simulink model "quad_new_leg_raibert_strategy_v2"  (R2018a)
settings: Solver=ode15s  StartTime=0.0  StopTime=10.0  RelTol=1e-3
values from neighbouring files (symbols this model uses):
  X = ([-L/2, L/2, L/2, -L/2])    [draw_cube.m]
  Y = ([-W/2, -W/2, W/2, W/2])    [draw_cube.m]
undefined symbols (not defined in the file or in its folder): body, ctrl, ground, planner, Z
libraries: nesl_utility x73, sm_lib x41, simulink x29, Contact_Forces_Lib x4, Parts_Lib x4, sharedtransform x1, dspstat3 x1
(part 4 of 4)

== system quad_new_leg_raibert_strategy_v2/leg_rl/u_joint_ctrl  ==
  tgt_angle : Inport
  has_ctrl : Inport  Port=2
  PID Controller : simulink/Continuous/PID Controller  Controller=PID  TimeDomain=Continuous-time  SampleTime=-1  IntegratorMethod=Forward Euler  FilterMethod=Forward Euler  Form=Parallel  UseFilter=on  ControllerParametersSource=internal  P=ctrl.pos_kp  I=ctrl.pos_ki  D=ctrl.pos_kd  N=100  InitialConditionSource=internal  InitialConditionForIntegrator=0  InitialConditionForFilter=0  ExternalReset=none  LimitOutput=off  UpperSaturationLimit=inf  LowerSaturationLimit=-inf  LinearizeAsGain=on  AntiWindupMode=none  Kb=1  TrackingMode=off  Kt=1  PParamMin=[]  PParamMax=[]  IParamMin=[]  IParamMax=[]  DParamMin=[]  DParamMax=[]  NParamMin=[]  NParamMax=[]  KbParamMin=[]  KbParamMax=[]  KtParamMin=[]  KtParamMax=[]  POutMin=[]  POutMax=[]  IOutMin=[]  IOutMax=[]  DOutMin=[]  DOutMax=[]  NOutMin=[]  NOutMax=[]  KbOutMin=[]  KbOutMax=[]  KtOutMin=[]  KtOutMax=[]  IntegratorOutMin=[]  IntegratorOutMax=[]  FilterOutMin=[]  FilterOutMax=[]  SumOutMin=[]  SumOutMax=[]  SumI1OutMin=[]  SumI1OutMax=[]  SumI2OutMin=[]  SumI2OutMax=[]  SumI3OutMin=[]  SumI3OutMax=[]  SumDOutMin=[]  SumDOutMax=[]  SaturationOutMin=[]  SaturationOutMax=[]  IntegratorContinuousStateAttributes=''  IntegratorStateMustResolveToSignalObject=off  IntegratorRTWStateStorageClass=Auto  FilterContinuousStateAttributes=''  FilterStateMustResolveToSignalObject=off  FilterRTWStateStorageClass=Auto  DifferentiatorICPrevScaledInput=0  DifferentiatorOutMin=[]  DifferentiatorOutMax=[]  FilterDiffOutCoefMin=[]  FilterDiffOutCoefMax=[]  SumDenOutMin=[]  SumDenOutMax=[]  SumNumOutMin=[]  SumNumOutMax=[]  ReciprocalOutMin=[]  ReciprocalOutMax=[]  DivideOutMin=[]  DivideOutMax=[]  TunerSelectOption=Transfer Function Based (PID Tuner App)
  PID Controller3 : simulink/Continuous/PID Controller  Controller=PID  TimeDomain=Continuous-time  SampleTime=-1  IntegratorMethod=Forward Euler  FilterMethod=Forward Euler  Form=Parallel  UseFilter=on  ControllerParametersSource=internal  P=ctrl.vel_kp  I=ctrl.vel_ki  D=ctrl.vel_kd  N=100  InitialConditionSource=internal  InitialConditionForIntegrator=0  InitialConditionForFilter=0  ExternalReset=none  LimitOutput=off  UpperSaturationLimit=inf  LowerSaturationLimit=-inf  LinearizeAsGain=on  AntiWindupMode=none  Kb=1  TrackingMode=off  Kt=1  PParamMin=[]  PParamMax=[]  IParamMin=[]  IParamMax=[]  DParamMin=[]  DParamMax=[]  NParamMin=[]  NParamMax=[]  KbParamMin=[]  KbParamMax=[]  KtParamMin=[]  KtParamMax=[]  POutMin=[]  POutMax=[]  IOutMin=[]  IOutMax=[]  DOutMin=[]  DOutMax=[]  NOutMin=[]  NOutMax=[]  KbOutMin=[]  KbOutMax=[]  KtOutMin=[]  KtOutMax=[]  IntegratorOutMin=[]  IntegratorOutMax=[]  FilterOutMin=[]  FilterOutMax=[]  SumOutMin=[]  SumOutMax=[]  SumI1OutMin=[]  SumI1OutMax=[]  SumI2OutMin=[]  SumI2OutMax=[]  SumI3OutMin=[]  SumI3OutMax=[]  SumDOutMin=[]  SumDOutMax=[]  SaturationOutMin=[]  SaturationOutMax=[]  IntegratorContinuousStateAttributes=''  IntegratorStateMustResolveToSignalObject=off  IntegratorRTWStateStorageClass=Auto  FilterContinuousStateAttributes=''  FilterStateMustResolveToSignalObject=off  FilterRTWStateStorageClass=Auto  DifferentiatorICPrevScaledInput=0  DifferentiatorOutMin=[]  DifferentiatorOutMax=[]  FilterDiffOutCoefMin=[]  FilterDiffOutCoefMax=[]  SumDenOutMin=[]  SumDenOutMax=[]  SumNumOutMin=[]  SumNumOutMax=[]  ReciprocalOutMin=[]  ReciprocalOutMax=[]  DivideOutMin=[]  DivideOutMax=[]  TunerSelectOption=Transfer Function Based (PID Tuner App)
  PSConv3 : nesl_utility/PS-Simulink Converter  PhysicalDomain=network_engine_domain  SubClassName=ps_output  LeftPortType=input  RightPortType=output  PseudoPeriodic=off  Frequencies=[]  Unit=1  AffineConversion=off
  PSConv4 : nesl_utility/PS-Simulink Converter  PhysicalDomain=network_engine_domain  SubClassName=ps_output  LeftPortType=input  RightPortType=output  PseudoPeriodic=off  Frequencies=[]  Unit=1  AffineConversion=off
  Product : Product
  SPConv : nesl_utility/Simulink-PS Converter  PhysicalDomain=network_engine_domain  SubClassName=ps_input  LeftPortType=input  RightPortType=output  PseudoPeriodic=off  Frequencies=[]  NoiseDistribution=none  NoiseParameters=[]  Unit=1  AffineConversion=off  FilteringAndDerivatives=filter  SimscapeFilterOrder=2  InputFilterTimeConstant=0.001  UdotUserProvided=1
  Sum1 : Sum  Inputs=|+-
  Sum6 : Sum  Inputs=|+-
  curr_angle : PMIOPort  Side=Left
  curr_omega : PMIOPort  Port=2  Side=Left
  torque : PMIOPort  Port=3  Side=Right
  wires:
  tgt_angle/1 -> Sum1/1
  Sum1/1 -> PID Controller/1
  PID Controller/1 -> Sum6/1
  Sum6/1 -> PID Controller3/1
  Product/1 -> SPConv/1
  PSConv3/1 -> Sum1/2
  has_ctrl/1 -> Product/1
  PID Controller3/1 -> Product/2
  PSConv4/1 -> Sum6/2
  connections:
  PSConv3/LConn1 -- curr_angle/RConn1
  SPConv/RConn1 -- torque/RConn1
  curr_omega/RConn1 -- PSConv4/LConn1

== system quad_new_leg_raibert_strategy_v2/leg_rr/k_joint_ctrl ==
  tgt_angle : Inport
  has_ctrl : Inport  Port=2
  PID Controller : simulink/Continuous/PID Controller  Controller=PID  TimeDomain=Continuous-time  SampleTime=-1  IntegratorMethod=Forward Euler  FilterMethod=Forward Euler  Form=Parallel  UseFilter=on  ControllerParametersSource=internal  P=ctrl.pos_kp  I=ctrl.pos_ki  D=ctrl.pos_kd  N=100  InitialConditionSource=internal  InitialConditionForIntegrator=0  InitialConditionForFilter=0  ExternalReset=none  LimitOutput=off  UpperSaturationLimit=inf  LowerSaturationLimit=-inf  LinearizeAsGain=on  AntiWindupMode=none  Kb=1  TrackingMode=off  Kt=1  PParamMin=[]  PParamMax=[]  IParamMin=[]  IParamMax=[]  DParamMin=[]  DParamMax=[]  NParamMin=[]  NParamMax=[]  KbParamMin=[]  KbParamMax=[]  KtParamMin=[]  KtParamMax=[]  POutMin=[]  POutMax=[]  IOutMin=[]  IOutMax=[]  DOutMin=[]  DOutMax=[]  NOutMin=[]  NOutMax=[]  KbOutMin=[]  KbOutMax=[]  KtOutMin=[]  KtOutMax=[]  IntegratorOutMin=[]  IntegratorOutMax=[]  FilterOutMin=[]  FilterOutMax=[]  SumOutMin=[]  SumOutMax=[]  SumI1OutMin=[]  SumI1OutMax=[]  SumI2OutMin=[]  SumI2OutMax=[]  SumI3OutMin=[]  SumI3OutMax=[]  SumDOutMin=[]  SumDOutMax=[]  SaturationOutMin=[]  SaturationOutMax=[]  IntegratorContinuousStateAttributes=''  IntegratorStateMustResolveToSignalObject=off  IntegratorRTWStateStorageClass=Auto  FilterContinuousStateAttributes=''  FilterStateMustResolveToSignalObject=off  FilterRTWStateStorageClass=Auto  DifferentiatorICPrevScaledInput=0  DifferentiatorOutMin=[]  DifferentiatorOutMax=[]  FilterDiffOutCoefMin=[]  FilterDiffOutCoefMax=[]  SumDenOutMin=[]  SumDenOutMax=[]  SumNumOutMin=[]  SumNumOutMax=[]  ReciprocalOutMin=[]  ReciprocalOutMax=[]  DivideOutMin=[]  DivideOutMax=[]  TunerSelectOption=Transfer Function Based (PID Tuner App)
  PID Controller3 : simulink/Continuous/PID Controller  Controller=PID  TimeDomain=Continuous-time  SampleTime=-1  IntegratorMethod=Forward Euler  FilterMethod=Forward Euler  Form=Parallel  UseFilter=on  ControllerParametersSource=internal  P=ctrl.vel_kp  I=ctrl.vel_ki  D=ctrl.vel_kd  N=100  InitialConditionSource=internal  InitialConditionForIntegrator=0  InitialConditionForFilter=0  ExternalReset=none  LimitOutput=off  UpperSaturationLimit=inf  LowerSaturationLimit=-inf  LinearizeAsGain=on  AntiWindupMode=none  Kb=1  TrackingMode=off  Kt=1  PParamMin=[]  PParamMax=[]  IParamMin=[]  IParamMax=[]  DParamMin=[]  DParamMax=[]  NParamMin=[]  NParamMax=[]  KbParamMin=[]  KbParamMax=[]  KtParamMin=[]  KtParamMax=[]  POutMin=[]  POutMax=[]  IOutMin=[]  IOutMax=[]  DOutMin=[]  DOutMax=[]  NOutMin=[]  NOutMax=[]  KbOutMin=[]  KbOutMax=[]  KtOutMin=[]  KtOutMax=[]  IntegratorOutMin=[]  IntegratorOutMax=[]  FilterOutMin=[]  FilterOutMax=[]  SumOutMin=[]  SumOutMax=[]  SumI1OutMin=[]  SumI1OutMax=[]  SumI2OutMin=[]  SumI2OutMax=[]  SumI3OutMin=[]  SumI3OutMax=[]  SumDOutMin=[]  SumDOutMax=[]  SaturationOutMin=[]  SaturationOutMax=[]  IntegratorContinuousStateAttributes=''  IntegratorStateMustResolveToSignalObject=off  IntegratorRTWStateStorageClass=Auto  FilterContinuousStateAttributes=''  FilterStateMustResolveToSignalObject=off  FilterRTWStateStorageClass=Auto  DifferentiatorICPrevScaledInput=0  DifferentiatorOutMin=[]  DifferentiatorOutMax=[]  FilterDiffOutCoefMin=[]  FilterDiffOutCoefMax=[]  SumDenOutMin=[]  SumDenOutMax=[]  SumNumOutMin=[]  SumNumOutMax=[]  ReciprocalOutMin=[]  ReciprocalOutMax=[]  DivideOutMin=[]  DivideOutMax=[]  TunerSelectOption=Transfer Function Based (PID Tuner App)
  PSConv3 : nesl_utility/PS-Simulink Converter  PhysicalDomain=network_engine_domain  SubClassName=ps_output  LeftPortType=input  RightPortType=output  PseudoPeriodic=off  Frequencies=[]  Unit=1  AffineConversion=off
  PSConv4 : nesl_utility/PS-Simulink Converter  PhysicalDomain=network_engine_domain  SubClassName=ps_output  LeftPortType=input  RightPortType=output  PseudoPeriodic=off  Frequencies=[]  Unit=1  AffineConversion=off
  Product : Product
  SPConv : nesl_utility/Simulink-PS Converter  PhysicalDomain=network_engine_domain  SubClassName=ps_input  LeftPortType=input  RightPortType=output  PseudoPeriodic=off  Frequencies=[]  NoiseDistribution=none  NoiseParameters=[]  Unit=1  AffineConversion=off  FilteringAndDerivatives=filter  SimscapeFilterOrder=2  InputFilterTimeConstant=0.001  UdotUserProvided=1
  Sum1 : Sum  Inputs=|+-
  Sum6 : Sum  Inputs=|+-
  curr_angle : PMIOPort  Side=Left
  curr_omega : PMIOPort  Port=2  Side=Left
  torque : PMIOPort  Port=3  Side=Right
  wires:
  tgt_angle/1 -> Sum1/1
  Sum1/1 -> PID Controller/1
  PID Controller/1 -> Sum6/1
  Sum6/1 -> PID Controller3/1
  Product/1 -> SPConv/1
  PSConv3/1 -> Sum1/2
  has_ctrl/1 -> Product/1
  PID Controller3/1 -> Product/2
  PSConv4/1 -> Sum6/2
  connections:
  PSConv3/LConn1 -- curr_angle/RConn1
  SPConv/RConn1 -- torque/RConn1
  curr_omega/RConn1 -- PSConv4/LConn1

== system quad_new_leg_raibert_strategy_v2/leg_rr/s_joint_ctrl  ==
  tgt_angle : Inport
  has_ctrl : Inport  Port=2
  PID Controller : simulink/Continuous/PID Controller  Controller=PID  TimeDomain=Continuous-time  SampleTime=-1  IntegratorMethod=Forward Euler  FilterMethod=Forward Euler  Form=Parallel  UseFilter=on  ControllerParametersSource=internal  P=ctrl.pos_kp  I=ctrl.pos_ki  D=ctrl.pos_kd  N=100  InitialConditionSource=internal  InitialConditionForIntegrator=0  InitialConditionForFilter=0  ExternalReset=none  LimitOutput=off  UpperSaturationLimit=inf  LowerSaturationLimit=-inf  LinearizeAsGain=on  AntiWindupMode=none  Kb=1  TrackingMode=off  Kt=1  PParamMin=[]  PParamMax=[]  IParamMin=[]  IParamMax=[]  DParamMin=[]  DParamMax=[]  NParamMin=[]  NParamMax=[]  KbParamMin=[]  KbParamMax=[]  KtParamMin=[]  KtParamMax=[]  POutMin=[]  POutMax=[]  IOutMin=[]  IOutMax=[]  DOutMin=[]  DOutMax=[]  NOutMin=[]  NOutMax=[]  KbOutMin=[]  KbOutMax=[]  KtOutMin=[]  KtOutMax=[]  IntegratorOutMin=[]  IntegratorOutMax=[]  FilterOutMin=[]  FilterOutMax=[]  SumOutMin=[]  SumOutMax=[]  SumI1OutMin=[]  SumI1OutMax=[]  SumI2OutMin=[]  SumI2OutMax=[]  SumI3OutMin=[]  SumI3OutMax=[]  SumDOutMin=[]  SumDOutMax=[]  SaturationOutMin=[]  SaturationOutMax=[]  IntegratorContinuousStateAttributes=''  IntegratorStateMustResolveToSignalObject=off  IntegratorRTWStateStorageClass=Auto  FilterContinuousStateAttributes=''  FilterStateMustResolveToSignalObject=off  FilterRTWStateStorageClass=Auto  DifferentiatorICPrevScaledInput=0  DifferentiatorOutMin=[]  DifferentiatorOutMax=[]  FilterDiffOutCoefMin=[]  FilterDiffOutCoefMax=[]  SumDenOutMin=[]  SumDenOutMax=[]  SumNumOutMin=[]  SumNumOutMax=[]  ReciprocalOutMin=[]  ReciprocalOutMax=[]  DivideOutMin=[]  DivideOutMax=[]  TunerSelectOption=Transfer Function Based (PID Tuner App)
  PID Controller3 : simulink/Continuous/PID Controller  Controller=PID  TimeDomain=Continuous-time  SampleTime=-1  IntegratorMethod=Forward Euler  FilterMethod=Forward Euler  Form=Parallel  UseFilter=on  ControllerParametersSource=internal  P=ctrl.vel_kp  I=ctrl.vel_ki  D=ctrl.vel_kd  N=100  InitialConditionSource=internal  InitialConditionForIntegrator=0  InitialConditionForFilter=0  ExternalReset=none  LimitOutput=off  UpperSaturationLimit=inf  LowerSaturationLimit=-inf  LinearizeAsGain=on  AntiWindupMode=none  Kb=1  TrackingMode=off  Kt=1  PParamMin=[]  PParamMax=[]  IParamMin=[]  IParamMax=[]  DParamMin=[]  DParamMax=[]  NParamMin=[]  NParamMax=[]  KbParamMin=[]  KbParamMax=[]  KtParamMin=[]  KtParamMax=[]  POutMin=[]  POutMax=[]  IOutMin=[]  IOutMax=[]  DOutMin=[]  DOutMax=[]  NOutMin=[]  NOutMax=[]  KbOutMin=[]  KbOutMax=[]  KtOutMin=[]  KtOutMax=[]  IntegratorOutMin=[]  IntegratorOutMax=[]  FilterOutMin=[]  FilterOutMax=[]  SumOutMin=[]  SumOutMax=[]  SumI1OutMin=[]  SumI1OutMax=[]  SumI2OutMin=[]  SumI2OutMax=[]  SumI3OutMin=[]  SumI3OutMax=[]  SumDOutMin=[]  SumDOutMax=[]  SaturationOutMin=[]  SaturationOutMax=[]  IntegratorContinuousStateAttributes=''  IntegratorStateMustResolveToSignalObject=off  IntegratorRTWStateStorageClass=Auto  FilterContinuousStateAttributes=''  FilterStateMustResolveToSignalObject=off  FilterRTWStateStorageClass=Auto  DifferentiatorICPrevScaledInput=0  DifferentiatorOutMin=[]  DifferentiatorOutMax=[]  FilterDiffOutCoefMin=[]  FilterDiffOutCoefMax=[]  SumDenOutMin=[]  SumDenOutMax=[]  SumNumOutMin=[]  SumNumOutMax=[]  ReciprocalOutMin=[]  ReciprocalOutMax=[]  DivideOutMin=[]  DivideOutMax=[]  TunerSelectOption=Transfer Function Based (PID Tuner App)
  PSConv3 : nesl_utility/PS-Simulink Converter  PhysicalDomain=network_engine_domain  SubClassName=ps_output  LeftPortType=input  RightPortType=output  PseudoPeriodic=off  Frequencies=[]  Unit=1  AffineConversion=off
  PSConv4 : nesl_utility/PS-Simulink Converter  PhysicalDomain=network_engine_domain  SubClassName=ps_output  LeftPortType=input  RightPortType=output  PseudoPeriodic=off  Frequencies=[]  Unit=1  AffineConversion=off
  Product : Product
  SPConv : nesl_utility/Simulink-PS Converter  PhysicalDomain=network_engine_domain  SubClassName=ps_input  LeftPortType=input  RightPortType=output  PseudoPeriodic=off  Frequencies=[]  NoiseDistribution=none  NoiseParameters=[]  Unit=1  AffineConversion=off  FilteringAndDerivatives=filter  SimscapeFilterOrder=2  InputFilterTimeConstant=0.001  UdotUserProvided=1
  Sum1 : Sum  Inputs=|+-
  Sum6 : Sum  Inputs=|+-
  curr_angle : PMIOPort  Side=Left
  curr_omega : PMIOPort  Port=2  Side=Left
  torque : PMIOPort  Port=3  Side=Right
  wires:
  tgt_angle/1 -> Sum1/1
  Sum1/1 -> PID Controller/1
  PID Controller/1 -> Sum6/1
  Sum6/1 -> PID Controller3/1
  Product/1 -> SPConv/1
  PSConv3/1 -> Sum1/2
  has_ctrl/1 -> Product/1
  PID Controller3/1 -> Product/2
  PSConv4/1 -> Sum6/2
  connections:
  PSConv3/LConn1 -- curr_angle/RConn1
  SPConv/RConn1 -- torque/RConn1
  curr_omega/RConn1 -- PSConv4/LConn1

== system quad_new_leg_raibert_strategy_v2/leg_rr/u_joint_ctrl  ==
  tgt_angle : Inport
  has_ctrl : Inport  Port=2
  PID Controller : simulink/Continuous/PID Controller  Controller=PID  TimeDomain=Continuous-time  SampleTime=-1  IntegratorMethod=Forward Euler  FilterMethod=Forward Euler  Form=Parallel  UseFilter=on  ControllerParametersSource=internal  P=ctrl.pos_kp  I=ctrl.pos_ki  D=ctrl.pos_kd  N=100  InitialConditionSource=internal  InitialConditionForIntegrator=0  InitialConditionForFilter=0  ExternalReset=none  LimitOutput=off  UpperSaturationLimit=inf  LowerSaturationLimit=-inf  LinearizeAsGain=on  AntiWindupMode=none  Kb=1  TrackingMode=off  Kt=1  PParamMin=[]  PParamMax=[]  IParamMin=[]  IParamMax=[]  DParamMin=[]  DParamMax=[]  NParamMin=[]  NParamMax=[]  KbParamMin=[]  KbParamMax=[]  KtParamMin=[]  KtParamMax=[]  POutMin=[]  POutMax=[]  IOutMin=[]  IOutMax=[]  DOutMin=[]  DOutMax=[]  NOutMin=[]  NOutMax=[]  KbOutMin=[]  KbOutMax=[]  KtOutMin=[]  KtOutMax=[]  IntegratorOutMin=[]  IntegratorOutMax=[]  FilterOutMin=[]  FilterOutMax=[]  SumOutMin=[]  SumOutMax=[]  SumI1OutMin=[]  SumI1OutMax=[]  SumI2OutMin=[]  SumI2OutMax=[]  SumI3OutMin=[]  SumI3OutMax=[]  SumDOutMin=[]  SumDOutMax=[]  SaturationOutMin=[]  SaturationOutMax=[]  IntegratorContinuousStateAttributes=''  IntegratorStateMustResolveToSignalObject=off  IntegratorRTWStateStorageClass=Auto  FilterContinuousStateAttributes=''  FilterStateMustResolveToSignalObject=off  FilterRTWStateStorageClass=Auto  DifferentiatorICPrevScaledInput=0  DifferentiatorOutMin=[]  DifferentiatorOutMax=[]  FilterDiffOutCoefMin=[]  FilterDiffOutCoefMax=[]  SumDenOutMin=[]  SumDenOutMax=[]  SumNumOutMin=[]  SumNumOutMax=[]  ReciprocalOutMin=[]  ReciprocalOutMax=[]  DivideOutMin=[]  DivideOutMax=[]  TunerSelectOption=Transfer Function Based (PID Tuner App)
  PID Controller3 : simulink/Continuous/PID Controller  Controller=PID  TimeDomain=Continuous-time  SampleTime=-1  IntegratorMethod=Forward Euler  FilterMethod=Forward Euler  Form=Parallel  UseFilter=on  ControllerParametersSource=internal  P=ctrl.vel_kp  I=ctrl.vel_ki  D=ctrl.vel_kd  N=100  InitialConditionSource=internal  InitialConditionForIntegrator=0  InitialConditionForFilter=0  ExternalReset=none  LimitOutput=off  UpperSaturationLimit=inf  LowerSaturationLimit=-inf  LinearizeAsGain=on  AntiWindupMode=none  Kb=1  TrackingMode=off  Kt=1  PParamMin=[]  PParamMax=[]  IParamMin=[]  IParamMax=[]  DParamMin=[]  DParamMax=[]  NParamMin=[]  NParamMax=[]  KbParamMin=[]  KbParamMax=[]  KtParamMin=[]  KtParamMax=[]  POutMin=[]  POutMax=[]  IOutMin=[]  IOutMax=[]  DOutMin=[]  DOutMax=[]  NOutMin=[]  NOutMax=[]  KbOutMin=[]  KbOutMax=[]  KtOutMin=[]  KtOutMax=[]  IntegratorOutMin=[]  IntegratorOutMax=[]  FilterOutMin=[]  FilterOutMax=[]  SumOutMin=[]  SumOutMax=[]  SumI1OutMin=[]  SumI1OutMax=[]  SumI2OutMin=[]  SumI2OutMax=[]  SumI3OutMin=[]  SumI3OutMax=[]  SumDOutMin=[]  SumDOutMax=[]  SaturationOutMin=[]  SaturationOutMax=[]  IntegratorContinuousStateAttributes=''  IntegratorStateMustResolveToSignalObject=off  IntegratorRTWStateStorageClass=Auto  FilterContinuousStateAttributes=''  FilterStateMustResolveToSignalObject=off  FilterRTWStateStorageClass=Auto  DifferentiatorICPrevScaledInput=0  DifferentiatorOutMin=[]  DifferentiatorOutMax=[]  FilterDiffOutCoefMin=[]  FilterDiffOutCoefMax=[]  SumDenOutMin=[]  SumDenOutMax=[]  SumNumOutMin=[]  SumNumOutMax=[]  ReciprocalOutMin=[]  ReciprocalOutMax=[]  DivideOutMin=[]  DivideOutMax=[]  TunerSelectOption=Transfer Function Based (PID Tuner App)
  PSConv3 : nesl_utility/PS-Simulink Converter  PhysicalDomain=network_engine_domain  SubClassName=ps_output  LeftPortType=input  RightPortType=output  PseudoPeriodic=off  Frequencies=[]  Unit=1  AffineConversion=off
  PSConv4 : nesl_utility/PS-Simulink Converter  PhysicalDomain=network_engine_domain  SubClassName=ps_output  LeftPortType=input  RightPortType=output  PseudoPeriodic=off  Frequencies=[]  Unit=1  AffineConversion=off
  Product : Product
  SPConv : nesl_utility/Simulink-PS Converter  PhysicalDomain=network_engine_domain  SubClassName=ps_input  LeftPortType=input  RightPortType=output  PseudoPeriodic=off  Frequencies=[]  NoiseDistribution=none  NoiseParameters=[]  Unit=1  AffineConversion=off  FilteringAndDerivatives=filter  SimscapeFilterOrder=2  InputFilterTimeConstant=0.001  UdotUserProvided=1
  Sum1 : Sum  Inputs=|+-
  Sum6 : Sum  Inputs=|+-
  curr_angle : PMIOPort  Side=Left
  curr_omega : PMIOPort  Port=2  Side=Left
  torque : PMIOPort  Port=3  Side=Right
  wires:
  PSConv4/1 -> Sum6/2
  PID Controller3/1 -> Product/2
  has_ctrl/1 -> Product/1
  PSConv3/1 -> Sum1/2
  Product/1 -> SPConv/1
  Sum6/1 -> PID Controller3/1
  PID Controller/1 -> Sum6/1
  Sum1/1 -> PID Controller/1
  tgt_angle/1 -> Sum1/1
  connections:
  curr_omega/RConn1 -- PSConv4/LConn1
  SPConv/RConn1 -- torque/RConn1
  PSConv3/LConn1 -- curr_angle/RConn1

== matlab function quad_new_leg_raibert_strategy_v2/Controller/QuadCtrl ==
  settings: updateMethod=DISCRETE
  data: fl_ang input; tgt_ctrl_fl output; fr_ang input; rl_ang input; rr_ang input; contact_state input; body_R input; sensing_info input; tgt_ctrl_fr output; tgt_ctrl_rl output; tgt_ctrl_rr output; t input; body parameter; planner parameter; ctrl_state output; debug output
function [tgt_ctrl_fl,tgt_ctrl_fr,tgt_ctrl_rl,tgt_ctrl_rr, ctrl_state, debug] = ...
    controller(fl_ang, fr_ang, rl_ang, rr_ang, ...
    contact_state, body_R, sensing_info, t, body, planner)

% the sample time of the block is set to be 0.0025 (400Hz);
dt = 0.0025;
%unpack sensing_info
body_vx = sensing_info(4);
body_vy = sensing_info(5);

fl_ang_s = fl_ang(1); fl_ang_u = fl_ang(2); fl_ang_k = fl_ang(3);
fr_ang_s = fr_ang(1); fr_ang_u = fr_ang(2); fr_ang_k = fr_ang(3);
rl_ang_s = rl_ang(1); rl_ang_u = rl_ang(2); rl_ang_k = rl_ang(3);
rr_ang_s = rr_ang(1); rr_ang_u = rr_ang(2); rr_ang_k = rr_ang(3);
% forward kinematics
fl_end_effector = forward_kinematics(fl_ang_s, fl_ang_u, fl_ang_k, body); 
rl_end_effector = forward_kinematics(rl_ang_s, rl_ang_u, rl_ang_k, body);
fr_end_effector = forward_kinematics(fr_ang_s, fr_ang_u, fr_ang_k, body);
rr_end_effector = forward_kinematics(rr_ang_s, rr_ang_u, rr_ang_k, body); 

% distance from center of mass to shoulder
fl_offset = [body.shoulder_distance;body.y_length/2+body.shoulder_size/2;0];
fr_offset = [body.shoulder_distance;-body.y_length/2-body.shoulder_size/2;0];
rl_offset = [-body.shoulder_distance;body.y_length/2+body.shoulder_size/2;0];
rr_offset = [-body.shoulder_distance;-body.y_length/2-body.shoulder_size/2;0];

%virtual leg1 fl (front left) rr(rear right) body frame
curr_virtual_leg1 = (fl_end_effector + fl_offset + rr_end_effector + rr_offset)*0.5;
%virtual leg2 fr (front right) rl(rear left) body frame 
curr_virtual_leg2 = (fr_end_effector + fr_offset + rl_end_effector + rl_offset)*0.5;

%decide state and state transition helpers
persistent state;
persistent timer;
persistent timer2;
if isempty(state)
    state = 0;
end
if isempty(timer)
    timer = 0;
end
if isempty(timer2)
    timer2 = 0;
end

% init variables
           % fl fr rl rr
has_u_ctrl = [1 1 1 1];
normal_virtual_leg1 = [0;0;planner.stand_height];
normal_virtual_leg2 = [0;0;planner.stand_height];
move_fl_end_effector = normal_virtual_leg1;
move_rr_end_effector = normal_virtual_leg1;
move_fr_end_effector = normal_virtual_leg2;
move_rl_end_effector = normal_virtual_leg2;
     
% state machine 

if state == 0 % standby state
    % in this state, just do nothing, but use time to make sure that all
    % feet stands on the ground 
    if contact_state(1) == 1 && contact_state(2) == 1 && contact_state(3) == 1 && contact_state(4) == 1
        %all foot on ground
        if abs(body_vx) < planner.state0_vel_thres 
            timer = timer + 1;
        else
            timer = 0;
        end
        if timer > planner.state0_trans_thres 
            state = 1;
            timer = 0;
        end
    end
elseif state == 1 % swing whole body to get a inital velocity
    timer2 = timer2 + 1;
    move_theta = planner.state0_swing_ang*sin(2*pi/planner.state0_swing_T*timer2);
    move_leg_Rx = [cos(move_theta) 0 sin(move_theta);
        0 1 0;
        -sin(move_theta) 0 cos(move_theta)];
    tgt_virtual_leg1_b = move_leg_Rx*normal_virtual_leg1;
    tgt_virtual_leg2_b = move_leg_Rx*normal_virtual_leg2;
    move_fl_end_effector = tgt_virtual_leg1_b;
    move_rr_end_effector = tgt_virtual_leg1_b;
    move_fr_end_effector = tgt_virtual_leg2_b;
    move_rl_end_effector = tgt_virtual_leg2_b;
        
    if body_vx > planner.state12_trans_speed
        timer = timer + 1;
    else
        timer = 0;
    end
    if timer > 40  %(keep a velocity larger than 0.2 for 0.1s)
        state = 2;
        timer = 0;
        timer2 = 0;
    end
    
%%% consider body rotation
% normal_virtual_leg1 = [0;0;planner.stand_height];
% normal_virtual_leg2 = [0;0;planner.stand_height];
% move_fl_end_effector = body_R'*(normal_virtual_leg1+fl_offset)-fl_offset;
% if norm(move_fl_end_effector) > body.max_stretch
%     move_fl_end_effector = move_fl_end_effector/norm(move_fl_end_effector)*body.max_stretch;
% end
% move_rr_end_effector = body_R'*(normal_virtual_leg1+rr_offset)-rr_offset;
% if norm(move_rr_end_effector) > body.max_stretch
%     move_rr_end_effector = move_rr_end_effector/norm(move_rr_end_effector)*body.max_stretch;
% end
% move_fr_end_effector = body_R'*(normal_virtual_leg2+fr_offset)-fr_offset;
% if norm(move_fr_end_effector) > body.max_stretch
%     move_fr_end_effector = move_fr_end_effector/norm(move_fr_end_effector)*body.max_stretch;
% end
% move_rl_end_effector = body_R'*(normal_virtual_leg2+rl_offset)-rl_offset;
% if norm(move_rl_end_effector) > body.max_stretch
%     move_rl_end_effector = move_rl_end_effector/norm(move_rl_end_effector)*body.max_stretch;
% end

elseif state == 2 % stance virtual leg1, swing virtual leg2
    timer2 = timer2 + 1;
    if timer2 > planner.leg_swing_time %(0.5s finish movement)
        timer2 = planner.leg_swing_time;
    end
    % stance leg no u control but need to balance the body
               % fl fr rl rr
    has_u_ctrl = [0 1 1 0];
    stance_length_coeff = 0.97+0.03*(timer2/planner.leg_swing_time);
    tgt_virtual_leg1_b = stance_length_coeff*normal_virtual_leg1;
    move_fl_end_effector = tgt_virtual_leg1_b;
    move_rr_end_effector = tgt_virtual_leg1_b;
    
    
    % swing leg must consider body angle 
    t = timer2/planner.leg_swing_time;
%     move_theta = -11/180*pi*(t);
    length_coeff = 0.8*t^2-0.8*t+1;
    % move leg in x direction
    move_theta = get_move_angle(length_coeff*normal_virtual_leg2,body_vx, planner.tgt_body_vx, planner);
    move_leg_Rx = [cos(move_theta) 0 sin(move_theta);
        0 1 0;
        -sin(move_theta) 0 cos(move_theta)];
    tgt_virtual_leg2_b = length_coeff*move_leg_Rx*normal_virtual_leg2;
    % move leg in y direction
    sagittal_angle = get_sagittal_angle(tgt_virtual_leg2_b,body_R, body_vy, planner);
    move_leg_Ry =[1 0 0;
                 0 cos(sagittal_angle) -sin(sagittal_angle);
                 0 sin(sagittal_angle) cos(sagittal_angle)];
    tgt_virtual_leg2_b = move_leg_Ry*tgt_virtual_leg2_b;
    
    
    move_fr_end_effector = body_R'*(tgt_virtual_leg2_b+fr_offset)-fr_offset;
    if norm(move_fr_end_effector) > body.max_stretch
        move_fr_end_effector = move_fr_end_effector/norm(move_fr_end_effector)*body.max_stretch;
    end
    move_rl_end_effector = body_R'*(tgt_virtual_leg2_b+rl_offset)-rl_offset;
    if norm(move_rl_end_effector) > body.max_stretch
        move_rl_end_effector = move_rl_end_effector/norm(move_rl_end_effector)*body.max_stretch;
    end
    
    % state transition
%     if timer2 == planner.leg_swing_time
    if timer2 > 0.5*planner.leg_swing_time && contact_state(2) == 1 && contact_state(3) == 1
        timer = timer + 1;
    else
        timer = 0;
    end
    if timer > 5   % to be determined
        state = 3;
        timer = 0;
        timer2 = 0;
    end
    
elseif state == 3 % swing virtual leg1, stance virtual leg2
    timer2 = timer2 + 1;
    if timer2 > planner.leg_swing_time %(0.5s finish movement)
        timer2 = planner.leg_swing_time;
    end
    % stance leg no u control but need to balance the body
               % fl fr rl rr
    has_u_ctrl = [1 0 0 1];
    stance_length_coeff = 0.97+0.03*(timer2/planner.leg_swing_time);
    tgt_virtual_leg2_b = stance_length_coeff*normal_virtual_leg2;
    move_fr_end_effector = tgt_virtual_leg2_b;
    move_rl_end_effector = tgt_virtual_leg2_b;
    
    % swing leg must consider body angle 
    t = timer2/planner.leg_swing_time;
    % theta is a function of forward velocity 
%     move_theta = -11/180*pi*(t);
    length_coeff = 0.8*t^2-0.8*t+1;
    move_theta = get_move_angle(length_coeff*normal_virtual_leg1,body_vx, planner.tgt_body_vx, planner);
    move_leg_Rx = [cos(move_theta) 0 sin(move_theta);
        0 1 0;
        -sin(move_theta) 0 cos(move_theta)];
    tgt_virtual_leg1_b = length_coeff*move_leg_Rx*normal_virtual_leg1;
        % move leg in y direction
    sagittal_angle = get_sagittal_angle(tgt_virtual_leg1_b,body_R, body_vy, planner);
    move_leg_Ry =[1 0 0;
                 0 cos(sagittal_angle) -sin(sagittal_angle);
                 0 sin(sagittal_angle) cos(sagittal_angle)];
    tgt_virtual_leg1_b = move_leg_Ry*tgt_virtual_leg1_b;
    
    move_fl_end_effector = body_R'*(tgt_virtual_leg1_b+fl_offset)-fl_offset;
    if norm(move_fl_end_effector) > body.max_stretch
        move_fl_end_effector = move_fl_end_effector/norm(move_fl_end_effector)*body.max_stretch;
    end
    move_rr_end_effector = body_R'*(tgt_virtual_leg1_b+rr_offset)-rr_offset;
    if norm(move_rr_end_effector) > body.max_stretch
        move_rr_end_effector = move_rr_end_effector/norm(move_rr_end_effector)*body.max_stretch;
    end
    
    % state transition
%     if timer2 == planner.leg_swing_time
    if timer2 > 0.5*planner.leg_swing_time && contact_state(1) == 1 && contact_state(4) == 1
        timer = timer + 1;
    else
        timer = 0;
    end
    if timer > 5   % to be determined
        state = 2;
        timer = 0;
        timer2 = 0;
    end
end



% delta_ang = planner.swing_ang;
% move_theta1 = delta_ang*sin(2*pi/planner.time_circle*t);
% 
% debug = move_theta1;
% move_leg_y = [cos(move_theta1) 0 sin(move_theta1);
%                             0 1               0;
%              -sin(move_theta1) 0 cos(move_theta1)];
% tgt_virtual_leg1 = move_leg_y*normal_virtual_leg1;
% 
% tgt_virtual_leg2 = move_leg_y'*normal_virtual_leg2;
%          
% 
% move_fl_end_effector = body_R*tgt_virtual_leg1;
% move_rr_end_effector = body_R*tgt_virtual_leg1;
% move_fr_end_effector = body_R*tgt_virtual_leg2;
% move_rl_end_effector = body_R*tgt_virtual_leg2;

%% fl to joint
[inv_s,inv_u,inv_k] = inverse_kinematics(move_fl_end_effector, body);
fl_tgt_ang_s = inv_s; 
fl_tgt_ang_u = inv_u;       
fl_tgt_ang_k = inv_k; 
tgt_ctrl_fl = [fl_tgt_ang_s;fl_tgt_ang_u;fl_tgt_ang_k;has_u_ctrl(1)];

%% fr to joint
[inv_s,inv_u,inv_k] = inverse_kinematics(move_fr_end_effector, body);
fr_tgt_ang_s = inv_s;
fr_tgt_ang_u = inv_u;
fr_tgt_ang_k = inv_k;
tgt_ctrl_fr = [fr_tgt_ang_s;fr_tgt_ang_u;fr_tgt_ang_k;has_u_ctrl(2)];

%% rl to joint
[inv_s,inv_u,inv_k] = inverse_kinematics(move_rl_end_effector, body);
rl_tgt_ang_s = inv_s;
rl_tgt_ang_u = inv_u;
rl_tgt_ang_k = inv_k;
tgt_ctrl_rl = [rl_tgt_ang_s;rl_tgt_ang_u;rl_tgt_ang_k;has_u_ctrl(3)];

%% rr to joint
[inv_s,inv_u,inv_k] = inverse_kinematics(move_rr_end_effector, body);
rr_tgt_ang_s = inv_s;
rr_tgt_ang_u = inv_u;
rr_tgt_ang_k = inv_k; 
tgt_ctrl_rr = [rr_tgt_ang_s;rr_tgt_ang_u;rr_tgt_ang_k;has_u_ctrl(4)];

ctrl_state = state;
debug = timer;

end

function move_angle = get_move_angle(virtual_leg,body_vx, tgt_body_vx, planner)

    distance = body_vx* planner.Ts/2 + planner.Kv*(tgt_body_vx-body_vx);
    
    if distance > 0.5*norm(virtual_leg)
        distance = 0.5*norm(virtual_leg);
    elseif distance < -0.5*norm(virtual_leg)
        distance = -0.5*norm(virtual_leg);
    end
    
    move_angle = asin(distance/norm(virtual_leg));
    if move_angle > 20/180*pi
        move_angle = 20/180*pi;
    elseif move_angle < -20/180*pi
        move_angle = -20/180*pi;
    end
    
end

function move_angle = get_sagittal_angle(virtual_leg,body_R, body_vy, planner)

    distance = body_vy* planner.Ts/2 + planner.Kv*(0-body_vy);  
    % 2017-1-23 test, can move to 0.1, 0.2, 0.3 is not possible
    
    if distance > 0.5*norm(virtual_leg)
        distance = 0.5*norm(virtual_leg);
    elseif distance < -0.5*norm(virtual_leg)
        distance = -0.5*norm(virtual_leg);
    end
    
    move_angle = asin(distance/norm(virtual_leg));
    if move_angle > 20/180*pi
        move_angle = 20/180*pi;
    elseif move_angle < -20/180*pi
        move_angle = -20/180*pi;
    end
    
end
